simulink model "Robot_model_LPV_2DOFcontrol_fullSchedulingOrder_2DOF"  (R2013a)
settings: Solver=ode1  StartTime=0.0  StopTime=12  FixedStep=.001  RelTol=1e-3
StopFcn:
  | q1rms = rms(q1qr1.signals.values(:, 1) - q1qr1.signals.values(:, 2))
  | q2rms = rms(q2qr2.signals.values(:, 1) - q2qr2.signals.values(:, 2))
  | q3rms = rms(q3qr3.signals.values(:, 1) - q3qr3.signals.values(:, 2))
undefined symbols (not defined in the file or in its folder): inert, robot2DOFaffineLPVparamsA, theta_mid, theta_range, Xdsim
undefined symbols (not defined in the file): dKLFR_sim
libraries: simulink x1, dspmtrx3 x1
settings Model: Creator=Administrator  LastModifiedBy=Christian Hoffmann
settings DataIOCC: LimitDataPoints=off  SignalLoggingSaveFormat=ModelDataLogs  SaveOutput=off  SaveTime=off
settings OptimizationCC: ExpressionDepthLimit=2147483647  InitFltsAndDblsToZero=on
settings DebuggingCC: SaveWithParameterizedLinksMsg=none  SignalResolutionControl=TryResolveAllWithWarning  SolverPrmCheckMsg=none  MultiTaskDSMMsg=warning  MultiTaskCondExecSysMsg=none  FcnCallInpInsideContextMsg=UseLocalSettings  StrictBusMsg=Warning
settings HardwareCC: TargetUnknown=on
settings SFSimCC: SimParseCustomCode=off
settings RTWCC: IncludeERTFirstTime=on
settings GRTTargetCC: TargetFcnLib=ansi_tfl_tmw.mat  CombineOutputUpdateFcns=off  GRTInterface=on

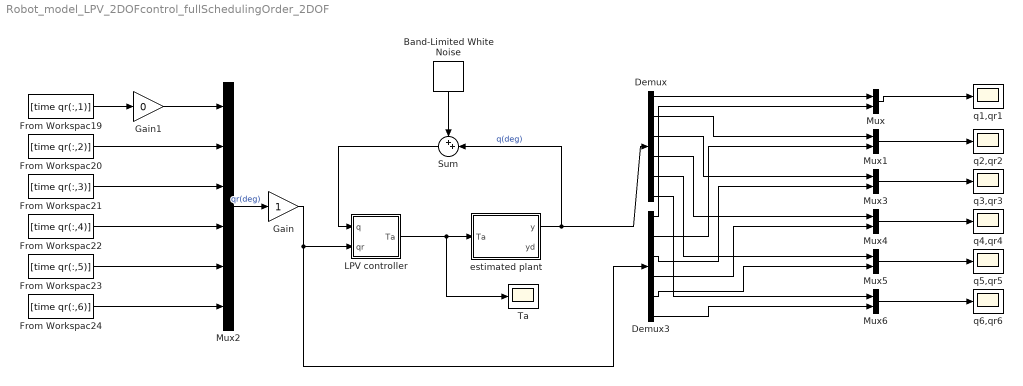
== system Robot_model_LPV_2DOFcontrol_fullSchedulingOrder_2DOF ==
  Band-Limited White Noise : simulink/Sources/Band-Limited White Noise  Cov=[0.000000001]  Ts=0.001  seed=[23341]
  Demux : Demux  Outputs=6
  Demux3 : Demux  Outputs=6
  From Workspac19 : FromWorkspace  VariableName=[time qr(:,1)]  SampleTime=0
  From Workspac20 : FromWorkspace  VariableName=[time qr(:,2)]  SampleTime=0
  From Workspac21 : FromWorkspace  VariableName=[time qr(:,3)]  SampleTime=0
  From Workspac22 : FromWorkspace  VariableName=[time qr(:,4)]  SampleTime=0
  From Workspac23 : FromWorkspace  VariableName=[time qr(:,5)]  SampleTime=0
  From Workspac24 : FromWorkspace  VariableName=[time qr(:,6)]  SampleTime=0
  Gain : Gain
  Gain1 : Gain  Gain=0
  LPV controller : Subsystem
  Mux{,1,3..6} (6 alike) : Mux  Inputs=2
  Mux2 : Mux  Inputs=6
  Sum : Sum  Inputs=++|
  Ta : Scope
      settings: YMin=-2.5  YMax=3  SaveName=ScopeData6
  estimated plant : Subsystem
  q1,qr1 : Scope
      settings: YMin=-33  YMax=-19  SaveName=q1qr1
  q2,qr2 : Scope
      settings: YMin=6.25  YMax=10.75  SaveName=q2qr2
  q3,qr3 : Scope
      settings: YMin=-9  YMax=14  SaveName=q3qr3
  q4,qr4 : Scope
      settings: YMin=0  YMax=375  SaveName=ScopeData3
  q5,qr5 : Scope
      settings: YMin=-50  YMax=50  SaveName=ScopeData4
  q6,qr6 : Scope
      settings: YMin=-60  YMax=45  SaveName=ScopeData5
  wires:
  Mux2/1 -> Gain/1  "qr(deg)"
  Demux/1 -> Mux/1
  Demux/2 -> Mux1/1
  Demux/3 -> Mux3/1
  Demux/4 -> Mux4/1
  Demux/5 -> Mux5/1
  Demux/6 -> Mux6/1
  Demux3/6 -> Mux6/2
  Demux3/5 -> Mux5/2
  Demux3/4 -> Mux4/2
  Demux3/3 -> Mux3/2
  Demux3/2 -> Mux1/2
  Demux3/1 -> Mux/2
  Mux/1 -> q1,qr1/1
  Mux1/1 -> q2,qr2/1
  Mux3/1 -> q3,qr3/1
  Mux4/1 -> q4,qr4/1
  Mux5/1 -> q5,qr5/1
  Mux6/1 -> q6,qr6/1
  LPV controller/1(Ta) -> Ta/1, estimated plant/1(Ta)
  From Workspac22/1 -> Mux2/4
  From Workspac23/1 -> Mux2/5
  From Workspac24/1 -> Mux2/6
  Gain/1 -> LPV controller/2(qr), Demux3/1
  From Workspac19/1 -> Gain1/1
  From Workspac20/1 -> Mux2/2
  From Workspac21/1 -> Mux2/3
  estimated plant/1(y) -> Sum/2, Demux/1  "q(deg)"
  Sum/1 -> LPV controller/1(q)
  Gain1/1 -> Mux2/1
  Band-Limited White Noise/1 -> Sum/1

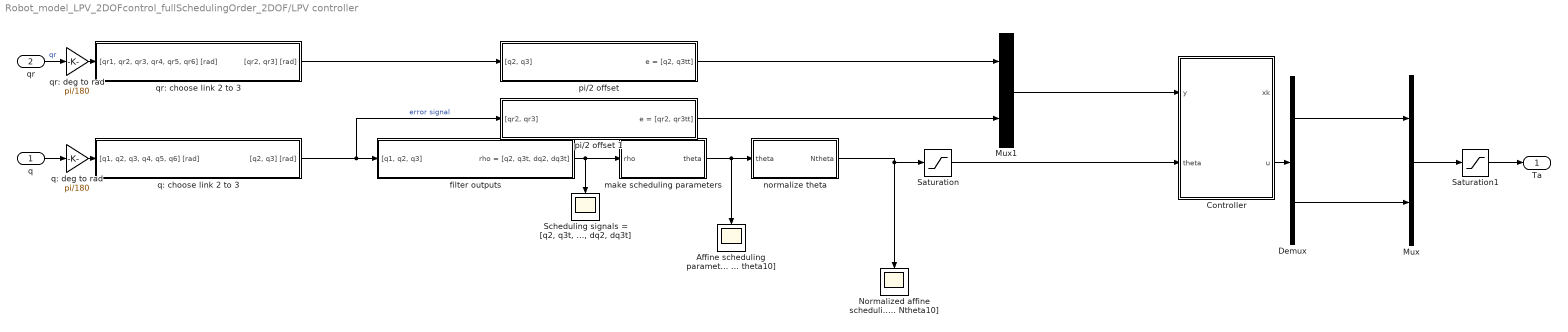
== system Robot_model_LPV_2DOFcontrol_fullSchedulingOrder_2DOF/LPV controller ==
  q : Inport
  qr : Inport  Port=2
  Affine scheduling parameters theta = [theta1 ... theta10] : Scope
      settings: ShowLegends=on
  Controller : Subsystem  mask{P=dKLFR_sim}
      mask prompts: P "Plant"
      mask Display:
      | port_label('output', 1, 'xk')
      | port_label('output', 2, 'u')
      | port_label('input' , 1, 'e')
      | port_label('input' , 2, 'theta')
      | fprintf('Controller')
  Demux : Demux  Outputs=2
  Mux : Mux  Inputs=2
  Mux1 : Mux  Inputs=2
  Normalized affine scheduling parameters Ntheta = [Ntheta1 ... Ntheta10] : Scope
      settings: YMin=-1.75  YMax=1.25
  Saturation : Saturate  UpperLimit=1  LowerLimit=-1
  Saturation1 : Saturate  UpperLimit=5  LowerLimit=-5
  "Scheduling signals = [q2, q3t, dq1, dq2, dq3t]" : Scope
      settings: SaveName=ScopeData2
  filter outputs : Subsystem
  make scheduling parameters : Subsystem
  normalize theta : Subsystem
  "pi/2 offset " : Subsystem
  pi/2 offset 1 : Subsystem
  q: choose link 2 to 3 : Subsystem
  q: deg to rad : Gain  Gain=pi/180
  qr: choose link 2 to 3 : Subsystem
  qr: deg to rad : Gain  Gain=pi/180
  Ta : Outport
  wires:
  q/1 -> q: deg to rad/1
  qr/1 -> qr: deg to rad/1  "qr"
  qr: choose link 2 to 3/1("[qr2, qr3] [rad]") -> "pi/2 offset "/1("[q2, q3]")
  q: deg to rad/1 -> q: choose link 2 to 3/1("[q1, q2, q3, q4, q5, q6] [rad]")
  qr: deg to rad/1 -> qr: choose link 2 to 3/1("[qr1, qr2, qr3, qr4, qr5, qr6] [rad]")
  q: choose link 2 to 3/1("[q2, q3] [rad]") -> filter outputs/1("[q1, q2, q3]"), pi/2 offset 1/1("[qr2, qr3]")  "error signal"
  Controller/2(u) -> Demux/1
  pi/2 offset 1/1("e = [qr2, qr3tt]") -> Mux1/2
  Mux1/1 -> Controller/1(y)
  Demux/1 -> Mux/1
  Demux/2 -> Mux/2
  normalize theta/1(Ntheta) -> Normalized affine scheduling parameters Ntheta = [Ntheta1 ... Ntheta10]/1, Saturation/1
  Mux/1 -> Saturation1/1
  "pi/2 offset "/1("e = [q2, q3tt]") -> Mux1/1
  Saturation/1 -> Controller/2(theta)
  filter outputs/1("rho = [q2, q3t, dq2, dq3t]") -> "Scheduling signals = [q2, q3t, dq1, dq2, dq3t]"/1, make scheduling parameters/1(rho)
  make scheduling parameters/1(theta) -> Affine scheduling parameters theta = [theta1 ... theta10]/1, normalize theta/1(theta)
  Saturation1/1 -> Ta/1

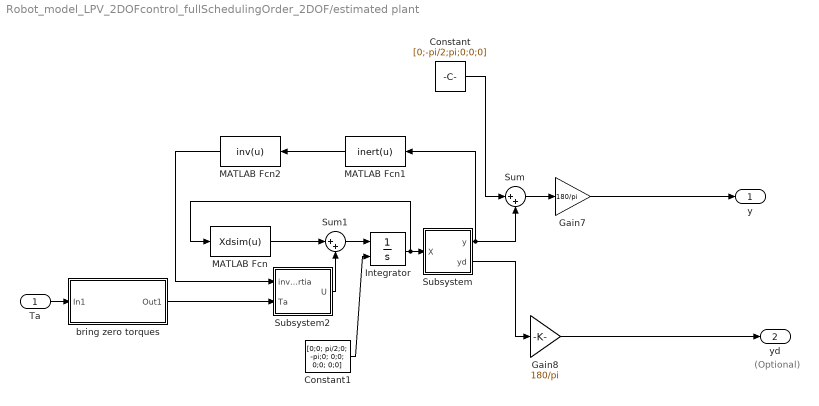
== system Robot_model_LPV_2DOFcontrol_fullSchedulingOrder_2DOF/estimated plant ==
  note: (Optional)
  Ta : Inport
  Constant : Constant  Value=[0;-pi/2;pi;0;0;0]
  Constant1 : Constant  Value="[0;0;    pi/2;0;    -pi;0;    0;0;    0;0;    0;0]"
      settings: AttributesFormatString=initial states, ready position
  Gain7 : Gain  Gain=180/pi
  Gain8 : Gain  Gain=180/pi
  Integrator : Integrator  InitialConditionSource=external
  MATLAB Fcn : MATLABFcn  MATLABFcn=Xdsim(u)
  MATLAB Fcn1 : MATLABFcn  MATLABFcn=inert(u)  Output1D=off
  MATLAB Fcn2 : MATLABFcn  MATLABFcn=inv(u)  Output1D=off
  Subsystem : Subsystem
  Subsystem2 : Subsystem
  Sum : Sum  Inputs=|++
  Sum1 : Sum  Inputs=|++
  bring zero torques : Subsystem
  y : Outport
  yd : Outport  Port=2
  wires:
  Sum/1 -> Gain7/1
  Constant/1 -> Sum/1
  Constant1/1 -> Integrator/2
  Integrator/1 -> MATLAB Fcn/1, Subsystem/1(X)
  Subsystem/2(yd) -> Gain8/1
  Subsystem/1(y) -> MATLAB Fcn1/1, Sum/2
  Sum1/1 -> Integrator/1
  MATLAB Fcn/1 -> Sum1/1
  Subsystem2/1("U ") -> Sum1/2
  MATLAB Fcn2/1 -> Subsystem2/1(inv inertia)
  Gain8/1 -> yd/1
  Gain7/1 -> y/1
  MATLAB Fcn1/1 -> MATLAB Fcn2/1
  Ta/1 -> bring zero torques/1(In1)
  bring zero torques/1(Out1) -> Subsystem2/2(Ta)

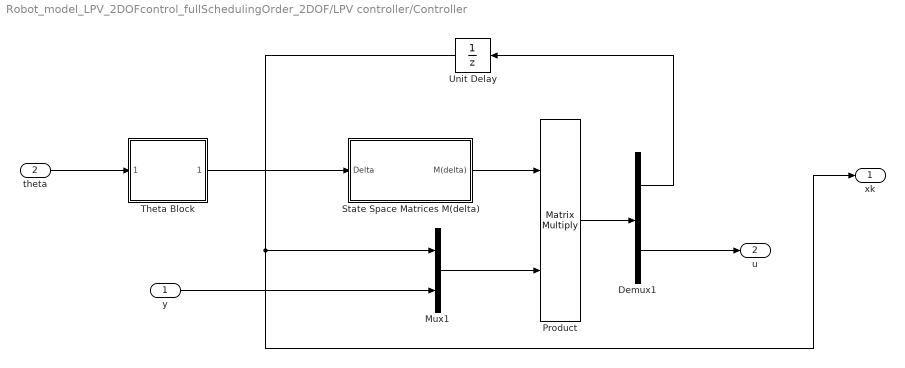
== system Robot_model_LPV_2DOFcontrol_fullSchedulingOrder_2DOF/LPV controller/Controller ==
  y : Inport
  theta : Inport  Port=2
  Demux1 : Demux  Outputs=[size(P.A, 1); size(P.C_y, 1)]
  Mux1 : Mux  Inputs=2
  Product : Product  Multiplication=Matrix(*)  RndMeth=Zero
  State Space Matrices M(delta) : Subsystem
  Theta Block : Subsystem
      mask Display:
      | patch([0.2 .5 0.8], [0.2 0.8 0.2], [0 0 0])
      | patch([0.25 .5 0.75], [0.25 0.75 0.25], [1 1 1])
  Unit Delay : UnitDelay  SampleTime=-1
  xk : Outport
  u : Outport  Port=2
  wires:
  y/1 -> Mux1/2
  Demux1/2 -> u/1
  Unit Delay/1 -> Mux1/1, xk/1
  Demux1/1 -> Unit Delay/1
  Product/1 -> Demux1/1
  Mux1/1 -> Product/2
  State Space Matrices M(delta)/1(M(delta)) -> Product/1
  theta/1 -> Theta Block/1(Scheduling Parameter Vector)
  Theta Block/1(Delta Block Vector) -> State Space Matrices M(delta)/1(Delta)

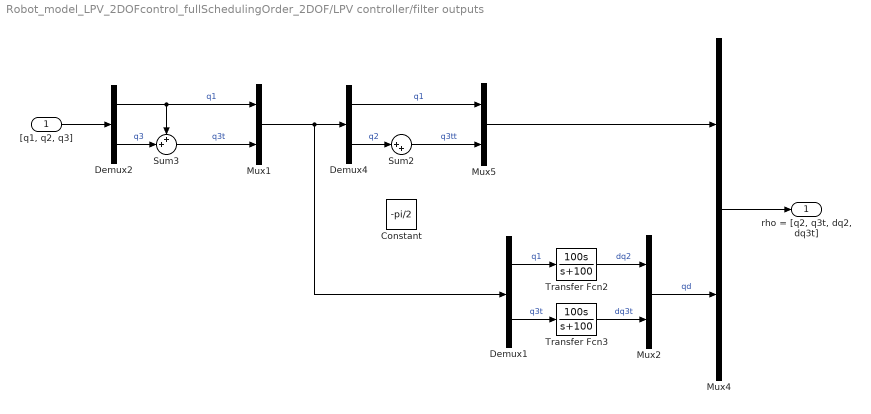
== system Robot_model_LPV_2DOFcontrol_fullSchedulingOrder_2DOF/LPV controller/filter outputs ==
  "[q1, q2, q3]" : Inport
  Constant : Constant  Value=-pi/2
  Demux1 : Demux  Outputs=2
  Demux2 : Demux  Outputs=2
  Demux4 : Demux  Outputs=2
  Mux{1..2,4..5} (4 alike) : Mux  Inputs=2
  Sum2 : Sum  Inputs=|++
  Sum3 : Sum  Inputs=++|
  Transfer Fcn2 : TransferFcn  Numerator=[100 0]  Denominator=[1 100]
  Transfer Fcn3 : TransferFcn  Numerator=[100 0]  Denominator=[1 100]
  "rho = [q2, q3t, dq2, dq3t]" : Outport
  wires:
  "[q1, q2, q3]"/1 -> Demux2/1
  Mux2/1 -> Mux4/2  "qd"
  Mux4/1 -> "rho = [q2, q3t, dq2, dq3t]"/1
  Demux2/2 -> Sum3/2  "q3"
  Sum3/1 -> Mux1/2  "q3t"
  Mux1/1 -> Demux1/1, Demux4/1
  Sum2/1 -> Mux5/2  "q3tt"
  Mux5/1 -> Mux4/1
  Demux1/2 -> Transfer Fcn3/1  "q3t"
  Transfer Fcn3/1 -> Mux2/2  "dq3t"
  Transfer Fcn2/1 -> Mux2/1  "dq2"
  Demux4/2 -> Sum2/1  "q2"
  Demux2/1 -> Mux1/1, Sum3/1  "q1"
  Demux4/1 -> Mux5/1  "q1"
  Demux1/1 -> Transfer Fcn2/1  "q1"

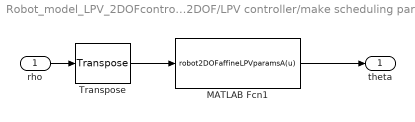
== system Robot_model_LPV_2DOFcontrol_fullSchedulingOrder_2DOF/LPV controller/make scheduling parameters ==
  rho : Inport
  MATLAB Fcn1 : MATLABFcn  MATLABFcn=robot2DOFaffineLPVparamsA(u)  Output1D=off
  Transpose : dspmtrx3/Transpose  Hermitian=off  overflowFlag=off
  theta : Outport
  wires:
  rho/1 -> Transpose/1
  MATLAB Fcn1/1 -> theta/1
  Transpose/1 -> MATLAB Fcn1/1

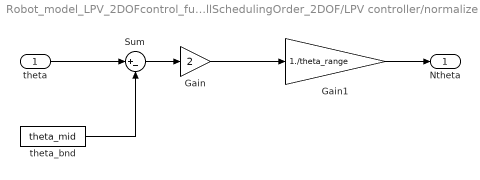
== system Robot_model_LPV_2DOFcontrol_fullSchedulingOrder_2DOF/LPV controller/normalize theta ==
  theta : Inport
  Gain : Gain  Gain=2
  Gain1 : Gain  Gain=1./theta_range
  Sum : Sum  Inputs=|+-
  theta_bnd : Constant  Value=theta_mid
  Ntheta : Outport
  wires:
  Gain1/1 -> Ntheta/1
  theta/1 -> Sum/1
  theta_bnd/1 -> Sum/2
  Sum/1 -> Gain/1
  Gain/1 -> Gain1/1

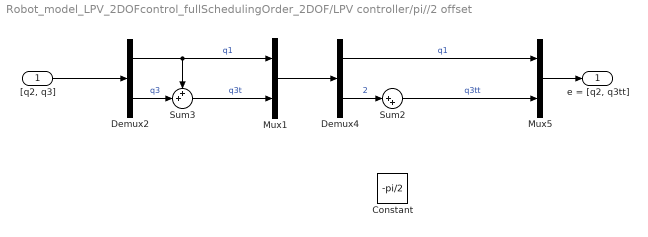
== system Robot_model_LPV_2DOFcontrol_fullSchedulingOrder_2DOF/LPV controller/pi//2 offset  ==
  "[q2, q3]" : Inport
  Constant : Constant  Value=-pi/2
  Demux2 : Demux  Outputs=2
  Demux4 : Demux  Outputs=2
  Mux1 : Mux  Inputs=2
  Mux5 : Mux  Inputs=2
  Sum2 : Sum  Inputs=|++
  Sum3 : Sum  Inputs=++|
  "e = [q2, q3tt]" : Outport
  wires:
  Mux1/1 -> Demux4/1
  Sum3/1 -> Mux1/2  "q3t"
  Demux2/2 -> Sum3/2  "q3"
  "[q2, q3]"/1 -> Demux2/1
  Mux5/1 -> "e = [q2, q3tt]"/1
  Demux4/2 -> Sum2/1  "2"
  Sum2/1 -> Mux5/2  "q3tt"
  Demux4/1 -> Mux5/1  "q1"
  Demux2/1 -> Sum3/1, Mux1/1  "q1"

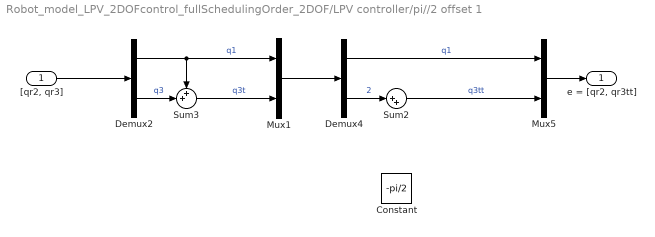
== system Robot_model_LPV_2DOFcontrol_fullSchedulingOrder_2DOF/LPV controller/pi//2 offset 1 ==
  "[qr2, qr3]" : Inport
  Constant : Constant  Value=-pi/2
  Demux2 : Demux  Outputs=2
  Demux4 : Demux  Outputs=2
  Mux1 : Mux  Inputs=2
  Mux5 : Mux  Inputs=2
  Sum2 : Sum  Inputs=|++
  Sum3 : Sum  Inputs=++|
  "e = [qr2, qr3tt]" : Outport
  wires:
  Demux2/1 -> Mux1/1, Sum3/1  "q1"
  Demux4/1 -> Mux5/1  "q1"
  Sum2/1 -> Mux5/2  "q3tt"
  Demux4/2 -> Sum2/1  "2"
  Mux5/1 -> "e = [qr2, qr3tt]"/1
  "[qr2, qr3]"/1 -> Demux2/1
  Demux2/2 -> Sum3/2  "q3"
  Sum3/1 -> Mux1/2  "q3t"
  Mux1/1 -> Demux4/1

== system Robot_model_LPV_2DOFcontrol_fullSchedulingOrder_2DOF/LPV controller/q: choose link 2 to 3 ==
  "[q1, q2, q3, q4, q5, q6] [rad]" : Inport
  Demux : Demux  Outputs=6
  Mux : Mux  Inputs=2
  "[q2, q3] [rad]" : Outport
  wires:
  "[q1, q2, q3, q4, q5, q6] [rad]"/1 -> Demux/1
  Mux/1 -> "[q2, q3] [rad]"/1
  Demux/2 -> Mux/1
  Demux/3 -> Mux/2

== system Robot_model_LPV_2DOFcontrol_fullSchedulingOrder_2DOF/LPV controller/qr: choose link 2 to 3 ==
  "[qr1, qr2, qr3, qr4, qr5, qr6] [rad]" : Inport
  Demux : Demux  Outputs=6
  Mux : Mux  Inputs=2
  "[qr2, qr3] [rad]" : Outport
  wires:
  "[qr1, qr2, qr3, qr4, qr5, qr6] [rad]"/1 -> Demux/1
  Mux/1 -> "[qr2, qr3] [rad]"/1
  Demux/3 -> Mux/2
  Demux/2 -> Mux/1

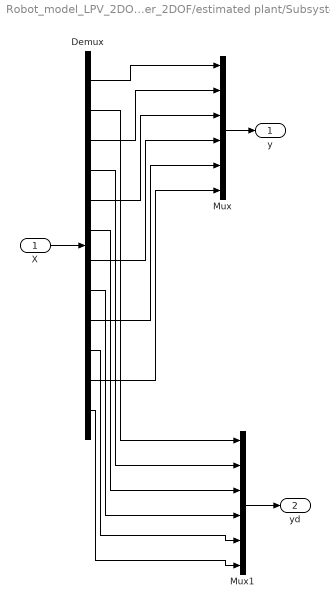
== system Robot_model_LPV_2DOFcontrol_fullSchedulingOrder_2DOF/estimated plant/Subsystem ==
  X : Inport
  Demux : Demux  Outputs=12
  Mux : Mux  Inputs=6
  Mux1 : Mux  Inputs=6
  y : Outport
  yd : Outport  Port=2
  wires:
  Demux/2 -> Mux1/1
  Demux/4 -> Mux1/2
  Demux/6 -> Mux1/3
  Demux/8 -> Mux1/4
  Demux/10 -> Mux1/5
  Demux/12 -> Mux1/6
  Demux/11 -> Mux/6
  Demux/9 -> Mux/5
  Demux/7 -> Mux/4
  Demux/5 -> Mux/3
  Demux/3 -> Mux/2
  Demux/1 -> Mux/1
  Mux/1 -> y/1
  Mux1/1 -> yd/1
  X/1 -> Demux/1

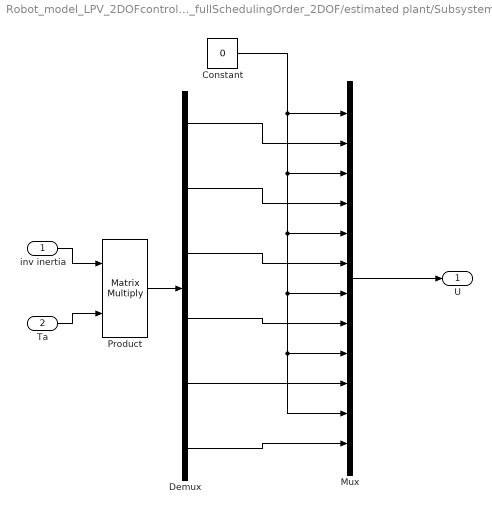
== system Robot_model_LPV_2DOFcontrol_fullSchedulingOrder_2DOF/estimated plant/Subsystem2 ==
  inv inertia : Inport
  Ta : Inport  Port=2
  Constant : Constant  Value=0
  Demux : Demux  Outputs=6
  Mux : Mux  Inputs=12
  Product : Product  Multiplication=Matrix(*)  RndMeth=Zero
  "U " : Outport
  wires:
  Constant/1 -> Mux/11, Mux/9, Mux/7, Mux/5, Mux/3, Mux/1
  Demux/6 -> Mux/12
  Demux/5 -> Mux/10
  Demux/4 -> Mux/8
  Demux/3 -> Mux/6
  Demux/2 -> Mux/4
  Demux/1 -> Mux/2
  Product/1 -> Demux/1
  Ta/1 -> Product/2
  inv inertia/1 -> Product/1
  Mux/1 -> "U "/1

== system Robot_model_LPV_2DOFcontrol_fullSchedulingOrder_2DOF/estimated plant/bring zero torques ==
  In1 : Inport
  Demux : Demux  Outputs=2
  Mux : Mux  Inputs=6
  Out1 : Outport
  wires:
  In1/1 -> Demux/1
  Mux/1 -> Out1/1
  Demux/2 -> Mux/3
  Demux/1 -> Mux/2

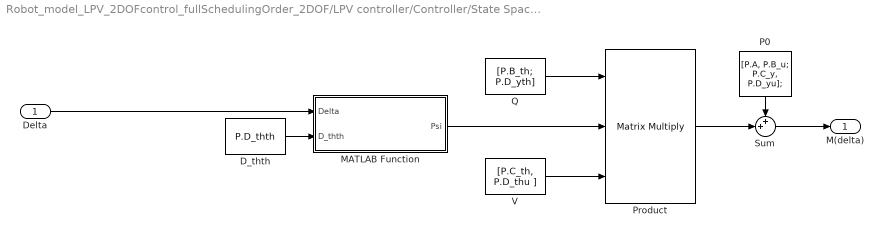
== system Robot_model_LPV_2DOFcontrol_fullSchedulingOrder_2DOF/LPV controller/Controller/State Space Matrices M(delta) ==
  Delta : Inport
  D_thth : Constant  Value=P.D_thth
  MATLAB Function : MATLAB Function  TreatAsAtomicUnit=on
  P0 : Constant  Value=[P.A, P.B_u; P.C_y, P.D_yu];  VectorParams1D=off
  Product : Product  Inputs=3  Multiplication=Matrix(*)  RndMeth=Zero
  Q : Constant  Value=[P.B_th; P.D_yth]
  Sum : Sum  Inputs=++|
  V : Constant  Value=[P.C_th, P.D_thu ]  VectorParams1D=off
  M(delta) : Outport
  wires:
  MATLAB Function/1(Psi) -> Product/2
  Delta/1 -> MATLAB Function/1(Delta)
  V/1 -> Product/3
  Sum/1 -> M(delta)/1
  P0/1 -> Sum/1
  Product/1 -> Sum/2
  Q/1 -> Product/1
  D_thth/1 -> MATLAB Function/2(D_thth)

== system Robot_model_LPV_2DOFcontrol_fullSchedulingOrder_2DOF/LPV controller/Controller/Theta Block ==
  Scheduling Parameter Vector : Inport
  Gain : Gain
  MATLAB Function : MATLAB Function  TreatAsAtomicUnit=on
  Delta Block Vector : Outport
  wires:
  MATLAB Function/1(Delta) -> Delta Block Vector/1
  Gain/1 -> MATLAB Function/1(DeltaVector)
  Scheduling Parameter Vector/1 -> Gain/1

== matlab function Robot_model_LPV_2DOFcontrol_fullSchedulingOrder_2DOF/LPV controller/Controller/Theta Block/MATLAB Function ==
  data: Delta output; DeltaVector input
function Delta = Delta(DeltaVector)
%#codegen
Delta = diag([ones(2, 1)*DeltaVector( 1); ...
              ones(1, 1)*DeltaVector( 2); ...
              ones(2, 1)*DeltaVector( 3); ...
              ones(1, 1)*DeltaVector( 4); ...
              ones(1, 1)*DeltaVector( 5); ...
              ones(1, 1)*DeltaVector( 6); ...
              ones(1, 1)*DeltaVector( 7); ...
              ones(1, 1)*DeltaVector( 8); ...
              ones(1, 1)*DeltaVector( 9); ...
              ones(1, 1)*DeltaVector(10)]);

== matlab function Robot_model_LPV_2DOFcontrol_fullSchedulingOrder_2DOF/LPV controller/Controller/State Space Matrices M(delta)/MATLAB Function ==
  data: Delta input; Psi output; D_thth input
function Psi = Psi(Delta, D_thth)
%#codegen

[nwth, nzth] = size(Delta);

Psi = Delta * (eye(nwth) - D_thth*Delta)^-1;
